simulink model "Feedbak_linearization"  (R2023a)
settings: Solver=VariableStepAuto  StartTime=0.0  StopTime=20  RelTol=1e-3
InitFcn:
  | FL_init
values from neighbouring files (symbols this model uses):
  At = 0.1257    [FL_init.m]
  Au = 0.0079    [FL_init.m]
  den = [0.00211600000000000,0.0920000000000000,1]    [FL_init.m]
  dz0 = 0    [FL_init.m]
  g = 9.81    [FL_init.m]    (also in INIT_R.m)
  h0 = 3    [FL_init.m]
  K = -0.1    [FL_init.m]
  Kv = 2    [FL_init.m]
  m = 0.261    [FL_init.m]    (also in INIT_R.m = 2)
  num = [1.39240000000000,2.36000000000000,1]    [FL_init.m]
  z0 = 0    [FL_init.m]
settings Model: Creator=rvitt  LastModifiedBy=rvitt

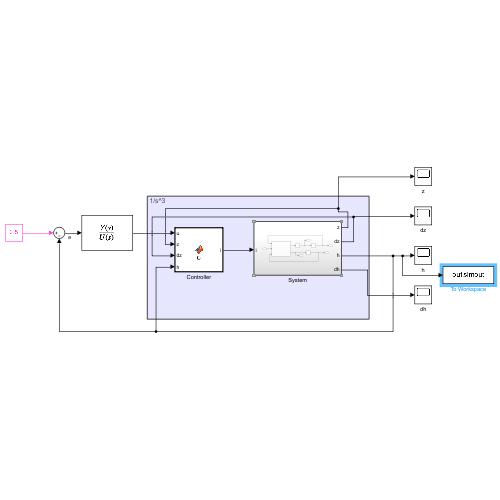
[thumbnail: Simulink's stored preview of the top-level diagram]
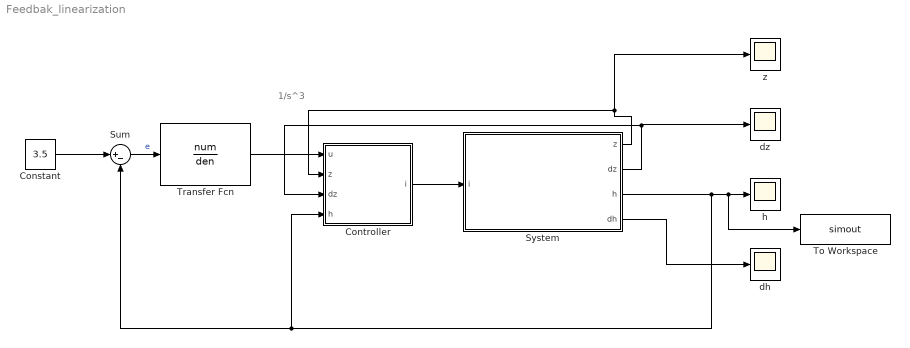
== system Feedbak_linearization ==
  note: 1/s^3
  Constant : Constant  Value=3.5
  Controller : MATLAB Function  TreatAsAtomicUnit=on
  Sum : Sum  Inputs=|+-
  System : Subsystem
  To Workspace : ToWorkspace  VariableName=simout  SaveFormat=Timeseries  SampleTime=-1
  Transfer Fcn : TransferFcn  Numerator=num  Denominator=den
  dh : Scope
  dz : Scope
  h : Scope
  z : Scope
  wires:
  System/1(z) -> z/1, Controller/2(z)
  System/2(dz) -> dz/1, Controller/3(dz)
  System/3(h) -> To Workspace/1, h/1, Controller/4(h), Sum/2
  System/4(dh) -> dh/1
  Constant/1 -> Sum/1
  Sum/1 -> Transfer Fcn/1  "e"
  Controller/1(i) -> System/1(i)
  Transfer Fcn/1 -> Controller/1(u)

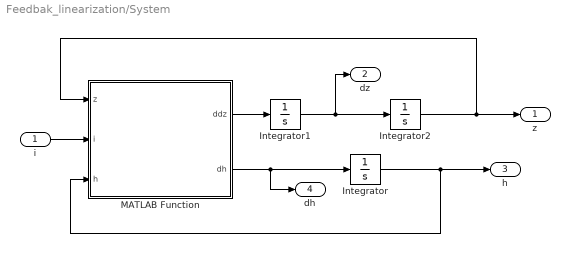
== system Feedbak_linearization/System ==
  i : Inport
  Integrator : Integrator  InitialCondition=h0
  Integrator1 : Integrator  InitialCondition=dz0
  Integrator2 : Integrator  InitialCondition=z0
  MATLAB Function : MATLAB Function  TreatAsAtomicUnit=on
  z : Outport
  dz : Outport  Port=2
  h : Outport  Port=3
  dh : Outport  Port=4
  wires:
  MATLAB Function/2(dh) -> Integrator/1, dh/1
  i/1 -> MATLAB Function/2(i)
  Integrator1/1 -> Integrator2/1, dz/1
  Integrator2/1 -> MATLAB Function/1(z), z/1
  Integrator/1 -> h/1, MATLAB Function/3(h)
  MATLAB Function/1(ddz) -> Integrator1/1

== matlab function Feedbak_linearization/Controller ==
  data: u input; z input; i output; dz input; h input; m parameter; Kv parameter; g parameter; Au parameter; K parameter; At parameter
function i = C(u, z ,dz, h, m, Kv, g, Au, K, At)

% State derivative
dh = Kv/At*(z-K) - Au/At*sqrt(2*g*h);

% Non linear function
% q = Au/At*sqrt(2*g)/2*(ddh/sqrt(h)+1/2*dh^2/h^(-3/2));

% H
p = Au/At^2*sqrt(2*g)/2*Kv*(dz/sqrt(h) - (z-K)/2*sqrt(h)*dh);
i = m*(1+9*z^2)/0.4*(g+At/Kv*p+At/Kv*u);

% Controller 
% q = Au/At^2*sqrt(2*g)/2*Kv*(dz/sqrt(h)-(z-K)/(2*h^(3/2)));
% i = m*(1+9*z^2)/0.4*(g + At/Kv*q + At/Kv*u);


% r = Au/At^2*sqrt(2*g)/2*Kv*(dz*sqrt(h)-(z-K)*1/2*dh/sqrt(h))/h;
% i = m*(1+9*z^2)/0.4*(g+ At/Kv*r+At/Kv*u);


% i = (1 + 9*z^2)/0.4*(m*g + Au*sqrt(2*g)/2 * ((Kv*dz)/(At*sqrt(h)) - (Au*sqrt(2*g)*dh)/(At*2*h) + dh^2/2*h^(-3/2)) + u);
%q = Au*sqrt(2*g)/2*(ddh/sqrt(h) + 1/2*dh^2/h^(-3/2));
%i = (1 + 9*z^2)/0.4*(m*g + q + u);

== matlab function Feedbak_linearization/System/MATLAB Function ==
  data: z input; i input; h input; ddz output; dh output; m parameter; Kv parameter; g parameter; Au parameter; K parameter; At parameter
function [ddz, dh] = model(z ,i, h, m, Kv, g, Au, K, At)

% System dynamics 
ddz = 0.4*i/(1 + 9*z^2)/m - g;
dh = Kv/At*(z-K) - Au/At*sqrt(2*g*h);


% ddh = Kv/At*dz - Au/At*sqrt(2*g)/2*dh/sqrt(h);
% 
% q = Au/At*sqrt(2*g)/2*(ddh/sqrt(h)+1/2*dh^2/h^(-3/2)); 
% y3 = Kv/At*(0.4/m*i/(1+9*z^2)-g)-q;
